simulink model "TS_forZS23"  (R2022b)
settings: Solver=ode45  StartTime=0.0  StopTime=10*60  RelTol=1e-3  EnableMultiTasking=on
undefined symbols (not defined in the file or in its folder): Advantech, PCI
libraries: sldrtlib x4
settings Model: Creator=Admin  LastModifiedBy=admin
settings SolverCC: AlgebraicLoopSolver=TrustRegion
settings DataIOCC: LimitDataPoints=on  SaveFormat=Array  ReturnWorkspaceOutputs=off
settings OptimizationCC: LifeSpan=inf
settings DebuggingCC: UnconnectedInputMsg=warning  UnconnectedOutputMsg=warning  UnconnectedLineMsg=warning  SFUnexpectedBacktrackingDiag=warning  SFNoUnconditionalDefaultTransitionDiag=warning  SFExecutionAtInitializationDiag=none  SFMachineParentedDataDiag=warning  ArithmeticOperatorsInVariantConditions=warning
settings HardwareCC: ProdBitPerPointer=32  ProdBitPerSizeT=32  ProdBitPerPtrDiffT=32  ProdLargestAtomicFloat=None  ProdIntDivRoundTo=Undefined  ProdEndianess=Unspecified  ProdWordSize=32  ProdHWDeviceType=32-bit Generic
settings ModelReferenceCC: PropagateSignalLabelsOutOfModel=off
settings SFSimCC: SimUseLocalCustomCode=off  CustomCodeUndefinedFunction=UseInterfaceOnly
settings RTWCC: RTWUseLocalCustomCode=off
settings CodeAppCC: StateflowObjectComments=on
settings GRTTargetCC: TargetLangStandard=C89/C90 (ANSI)
settings ConfigComp: CovMetricSettings=dw  CovSaveCumulativeToWorkspaceVar=on  CovSaveSingleToWorkspaceVar=on  CovExternalEMLEnable=off

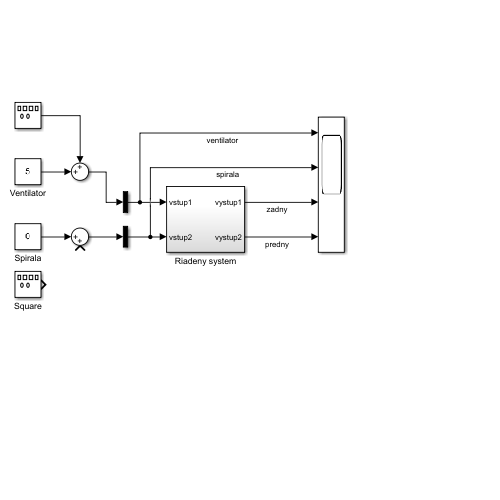
[thumbnail: Simulink's stored preview of the top-level diagram]
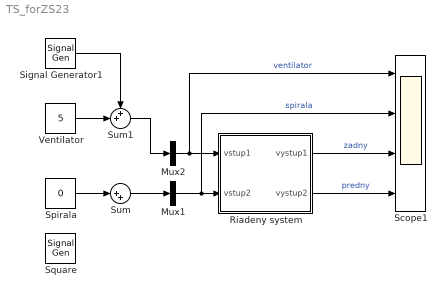
== system TS_forZS23 ==
  Mux1 : Mux  Inputs=1
  Mux2 : Mux  Inputs=1
  Riadeny system : Subsystem
  Scope1 : Scope  NumInputPorts=4
  Signal Generator1 : SignalGenerator  Frequency=1/20
  Spirala : Constant  Value=0
  Square : SignalGenerator  WaveForm=square  Amplitude=2  Frequency=1/40
  Sum : Sum  Inputs=|++
  Sum1 : Sum  Inputs=++|
  Ventilator : Constant  Value=5
  wires:
  Spirala/1 -> Sum/1
  Sum/1 -> Mux1/1
  Mux2/1 -> Scope1/1, Riadeny system/1(vstup1)  "ventilator"
  Riadeny system/1(vystup1) -> Scope1/3  "zadny"
  Riadeny system/2(vystup2) -> Scope1/4  "predny"
  Mux1/1 -> Scope1/2, Riadeny system/2(vstup2)  "spirala"
  Ventilator/1 -> Sum1/2
  Sum1/1 -> Mux2/1
  Signal Generator1/1 -> Sum1/1

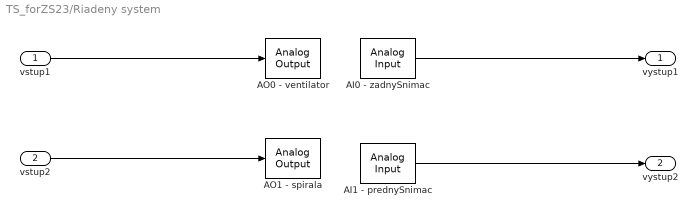
== system TS_forZS23/Riadeny system ==
  vstup1 : Inport
  vstup2 : Inport  Port=2
  AI0 - zadnySnimac : sldrtlib/Analog Input  SampleTime=0.1  MaxMissedTicks=10  ShowMissedTicks=off  YieldWhenWaiting=off  DrvName=Advantech/PCI-1711  DrvAddress=4294967295  DrvOptions=zeros(1,0)  Channels=1  RangeMode=1  VoltRange=1  DataType=1
      settings: AttributesFormatString=Advantech\nPCI-1711 [auto]
  AI1 - prednySnimac : sldrtlib/Analog Input  SampleTime=0.1  MaxMissedTicks=10  ShowMissedTicks=off  YieldWhenWaiting=off  DrvName=Advantech/PCI-1711  DrvAddress=4294967295  DrvOptions=zeros(1,0)  Channels=2  RangeMode=1  VoltRange=1  DataType=1
      settings: AttributesFormatString=Advantech\nPCI-1711 [auto]
  AO0 - ventilator : sldrtlib/Analog Output  SampleTime=0.1  MaxMissedTicks=10  ShowMissedTicks=off  YieldWhenWaiting=off  DrvName=Advantech/PCI-1711  DrvAddress=4294967295  DrvOptions=zeros(1,0)  Channels=1  RangeMode=1  VoltRange=2  InitialValue=[]  FinalValue=[]
      settings: AttributesFormatString=Advantech\nPCI-1711 [auto]
  AO1 - spirala : sldrtlib/Analog Output  SampleTime=0.1  MaxMissedTicks=10  ShowMissedTicks=off  YieldWhenWaiting=off  DrvName=Advantech/PCI-1711  DrvAddress=4294967295  DrvOptions=zeros(1,0)  Channels=2  RangeMode=1  VoltRange=2  InitialValue=[]  FinalValue=[]
      settings: AttributesFormatString=Advantech\nPCI-1711 [auto]
  vystup1 : Outport
  vystup2 : Outport  Port=2
  wires:
  vstup1/1 -> AO0 - ventilator/1
  vstup2/1 -> AO1 - spirala/1
  AI1 - prednySnimac/1 -> vystup2/1
  AI0 - zadnySnimac/1 -> vystup1/1
